simulink model "FSO_DEFINITIVO_700m - copia"  (R2025b)
settings: Solver=VariableStepAuto  StartTime=0.0  StopTime=0.0001  RelTol=1e-3
values from neighbouring files (symbols this model uses):
  bit_rate_bps = bit_rate_Gbps * 1e9    (= 1000000000)    [FSO_CALCULADORA_700m - copia.m]
  Pt_W = 10^((Pt_dBm - 30)/10)    (= 0.01)    [FSO_CALCULADORA_700m - copia.m]
  sigma_lnI_turb = sqrt(sigma_R2_turb)    [FSO_CALCULADORA_700m - copia.m]
  thr_opt_1 = thr_1 * correction_factor    [FSO_CALCULADORA_700m - copia.m]
  thr_opt_2 = thr_2 * correction_factor    [FSO_CALCULADORA_700m - copia.m]
  thr_opt_3 = thr_3 * correction_factor    [FSO_CALCULADORA_700m - copia.m]
  thr_opt_4 = thr_4 * correction_factor    [FSO_CALCULADORA_700m - copia.m]
undefined symbols (not defined in the file or in its folder): gain_clear, gain_extreme, gain_rain_mod, gain_turb
libraries: commrandsrc3 x1, commsink2 x1, commchan3 x1
settings Model: Creator=luigg  LastModifiedBy=luigg

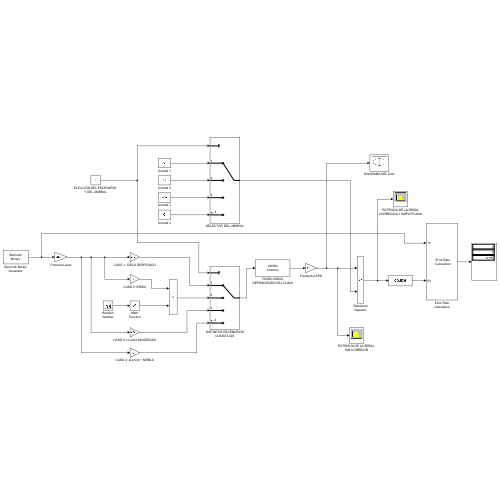
[thumbnail: Simulink's stored preview of the top-level diagram]
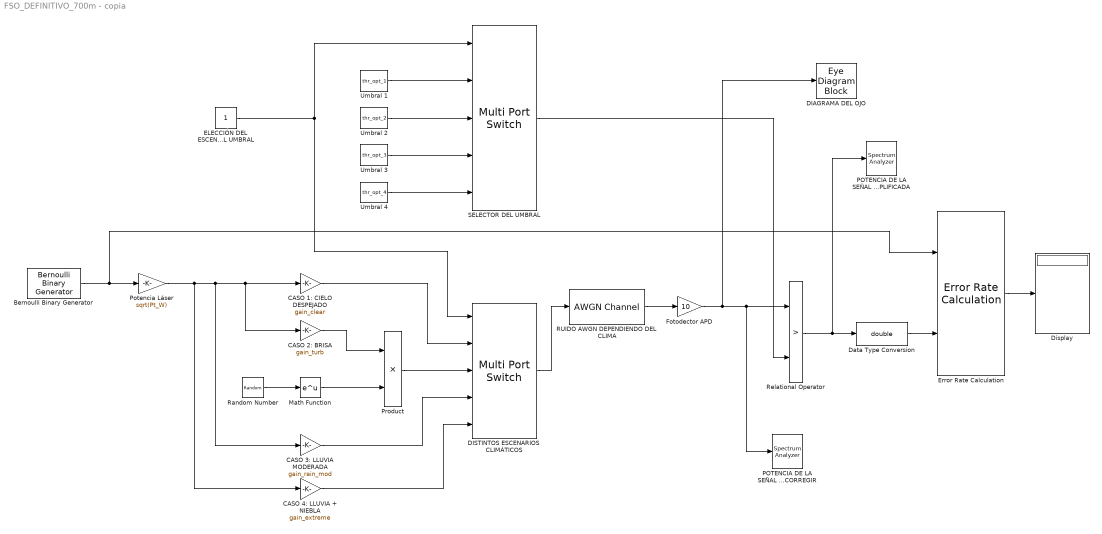
== system FSO_DEFINITIVO_700m - copia ==
  Bernoulli Binary Generator : commrandsrc3/Bernoulli Binary Generator  ProbabilityOfZero=0.5  SeedSource=Auto  Seed=0  SampleTime=1/bit_rate_bps  SamplesPerFrame=1  OutputDataType=double  SimulateUsing=Interpreted execution
  CASO 1: CIELO DESPEJADO : Gain  Gain=gain_clear
  CASO 2: BRISA : Gain  Gain=gain_turb
  CASO 3: LLUVIA MODERADA : Gain  Gain=gain_rain_mod
  CASO 4: LLUVIA + NIEBLA : Gain  Gain=gain_extreme
  DIAGRAMA DEL OJO : EyeDiagramBlock  WindowPosition=[517.000000,96.000000,662.000000,600.000000,]  Visible=on  ScopeFrameLocation=window  SamplesPerSymbol=1
  DISTINTOS ESCENARIOS CLIMÁTICOS : MultiPortSwitch  Inputs=4  SaturateOnIntegerOverflow=off  InputSameDT=off
  Data Type Conversion : DataTypeConversion  OutDataTypeStr=double  SaturateOnIntegerOverflow=off  RndMeth=Floor
  Display : Display
  ELECCIÓN DEL ESCENARIO Y DEL UMBRAL : Constant
  Error Rate Calculation : commsink2/Error Rate Calculation  N=0  st_delay=0  cp_mode=Entire frame  subframe=[]  PMode=Port  WsName=ErrorVec  RsMode2=off  stop=off  numErr=100  maxBits=1e6
  Fotodector APD : Gain  Gain=10
  Math Function : Math
  POTENCIA DE LA SEÑAL CORREGIDA Y AMPLIFICADA : SpectrumAnalyzer  WindowPosition=[369.000000,235.000000,798.000000,394.000000,]  Visible=on  ScopeFrameLocation=window  WindowInvariantSamplesPerUpdate=on  Span=999999999.9999999  StartFrequency=-499999999.99999994  StopFrequency=499999999.99999994  YLimits=[-13.728 28.0091]  SelectedToolstripTab=spectrumAnalyzerToolstrip.spectrumTab
  "POTENCIA DE LA SEÑAL SIN CORREGIR " : SpectrumAnalyzer  WindowPosition=[368.000000,182.000000,800.000000,500.000000,]  Visible=on  ScopeFrameLocation=window  WindowInvariantSamplesPerUpdate=on  Span=999999999.9999999  StartFrequency=-499999999.99999994  StopFrequency=499999999.99999994  YLimits=[-18.281 23.5162]
  Potencia Láser : Gain  Gain=sqrt(Pt_W)
  Product : Product
  RUIDO AWGN DEPENDIENDO DEL CLIMA : commchan3/AWGN Channel  LegacyMode=off  NoiseMethod="Signal to noise ratio  (Eb/No)"  noiseMode="Signal to noise ratio  (SNR)"  EbNo=30  EsNo=10  SNR=30  BitsPerSymbol=1  SignalPower=SigPow_1  SpecifySymbolPeriod=on  SamplesPerSymbol=1  SymbolPeriod=1/bit_rate_bps  VarianceSource=Parameter  Variance=1  RandomStream=Global stream  Seed=67  SimulateUsing=Code generation
  Random Number : RandomNumber  Mean=-sigma_lnI_turb^2 / 2  Variance=sigma_lnI_turb^2  Seed=[12345]  SampleTime=1e-3
  Relational Operator : RelationalOperator  Operator=>  OutDataTypeStr=boolean  RndMeth=Simplest  InputSameDT=off
  SELECTOR DEL UMBRAL : MultiPortSwitch  Inputs=4  SaturateOnIntegerOverflow=off  InputSameDT=off
  Umbral 1 : Constant  Value=thr_opt_1
  Umbral 2 : Constant  Value=thr_opt_2
  Umbral 3 : Constant  Value=thr_opt_3
  Umbral 4 : Constant  Value=thr_opt_4
  wires:
  CASO 2: BRISA/1 -> Product/1
  Potencia Láser/1 -> CASO 4: LLUVIA + NIEBLA/1, CASO 3: LLUVIA MODERADA/1, CASO 2: BRISA/1, CASO 1: CIELO DESPEJADO/1
  Random Number/1 -> Math Function/1
  Math Function/1 -> Product/2
  ELECCIÓN DEL ESCENARIO Y DEL UMBRAL/1 -> DISTINTOS ESCENARIOS CLIMÁTICOS/1, SELECTOR DEL UMBRAL/1
  Product/1 -> DISTINTOS ESCENARIOS CLIMÁTICOS/3
  Umbral 1/1 -> SELECTOR DEL UMBRAL/2
  Umbral 2/1 -> SELECTOR DEL UMBRAL/3
  Umbral 3/1 -> SELECTOR DEL UMBRAL/4
  Umbral 4/1 -> SELECTOR DEL UMBRAL/5
  Bernoulli Binary Generator/1 -> Error Rate Calculation/1, Potencia Láser/1
  DISTINTOS ESCENARIOS CLIMÁTICOS/1 -> RUIDO AWGN DEPENDIENDO DEL CLIMA/1
  Error Rate Calculation/1 -> Display/1
  RUIDO AWGN DEPENDIENDO DEL CLIMA/1 -> Fotodector APD/1
  Data Type Conversion/1 -> Error Rate Calculation/2
  SELECTOR DEL UMBRAL/1 -> Relational Operator/2
  Relational Operator/1 -> POTENCIA DE LA SEÑAL CORREGIDA Y AMPLIFICADA/1, Data Type Conversion/1
  Fotodector APD/1 -> "POTENCIA DE LA SEÑAL SIN CORREGIR "/1, Relational Operator/1, DIAGRAMA DEL OJO/1
  CASO 3: LLUVIA MODERADA/1 -> DISTINTOS ESCENARIOS CLIMÁTICOS/4
  CASO 4: LLUVIA + NIEBLA/1 -> DISTINTOS ESCENARIOS CLIMÁTICOS/5
  CASO 1: CIELO DESPEJADO/1 -> DISTINTOS ESCENARIOS CLIMÁTICOS/2
